simulink model "esercizio2sim_controllore_ricostruttore"  (R2018a)
settings: Solver=VariableStepAuto  StartTime=0.0  StopTime=25  RelTol=1e-7
values from neighbouring files (symbols this model uses):
  A = [2 1 -1; -3 -2 -1; -1 1 -4]    [esercizio1mat.m]    (also in esercizio2mat.m = [0 1 0 0; esercizio3mat.m = [1 1 0; -5 -3 0; 2 3 -1])
  B = B(:, 1)    [esercizio2mat.m]
  C = C(1, :)    [esercizio2mat.m]
  D = D(1, 1)    [esercizio2mat.m]
  g = 9.81    [esercizio2mat.m]
  k = acker(A, -b, autovalori); disp(k)    [esercizio1mat.m]    (also in esercizio2mat.m = acker(A, -B, autov_controllore); disp(k))
  L = 1    [esercizio2mat.m]
  l = lT'; disp(l)    [esercizio1mat.m]    (also in esercizio2mat.m)
  m = 1    [esercizio2mat.m]
  M = 10    [esercizio2mat.m]
  x0 = [0 0 pi/3 .0]'    [esercizio2mat.m]
  xhat0 = x0 + [0.01 -0.02 -0.01 0.02]'    [esercizio2mat.m]
settings Model: Creator=Matteo  LastModifiedBy=Matteo

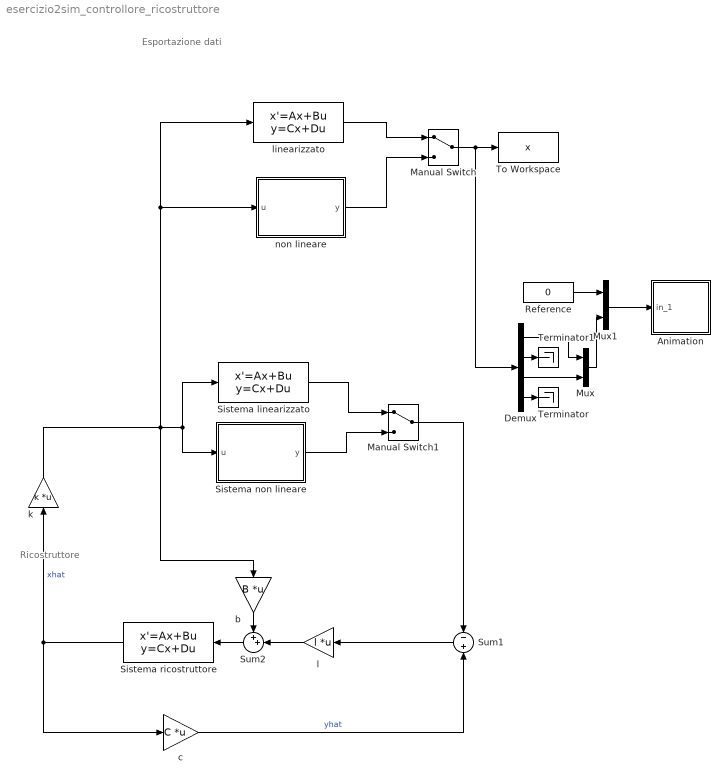
== system esercizio2sim_controllore_ricostruttore ==
  note: Esportazione dati
  note: Ricostruttore
  Animation : Subsystem  mask(Pendulum plot){RefBlock=Reference}
      mask prompts: RefBlock "DC reference signal block name:"
      mask help: Pendulum plot
      mask Help: Pendulum animation function using Handle graphics.
      mask Display: plot([-10 10],[0 0],[-2 -2 2 2],[0 1 1 0],[0 3],[1 5])
  Demux : Demux
  Manual Switch : ManualSwitch
  Manual Switch1 : ManualSwitch
  Mux : Mux  Inputs=2
  Mux1 : Mux  Inputs=2
  Reference : Constant  Value=0
  Sistema linearizzato : StateSpace  A=A  B=B  C=C  D=D  InitialCondition=x0
  Sistema non lineare : Subsystem
  Sistema ricostruttore : StateSpace  A=A  B=eye(4)  C=eye(4)  D=zeros(4)  InitialCondition=xhat0
  Sum1 : Sum  Inputs=-|+
  Sum2 : Sum  Inputs=++|
  Terminator : Terminator
  Terminator1 : Terminator
  To Workspace : ToWorkspace  VariableName=x  SaveFormat=Timeseries  SampleTime=0.05
  b : Gain  Gain=B  Multiplication=Matrix(K*u)
  c : Gain  Gain=C  Multiplication=Matrix(K*u)
  k : Gain  Gain=k  Multiplication=Matrix(K*u)
  l : Gain  Gain=l  Multiplication=Matrix(K*u)
  linearizzato : StateSpace  A=A  B=B  C=eye(4)  D=zeros(4,1)  InitialCondition=x0
  non lineare : Subsystem
  wires:
  Sistema ricostruttore/1 -> c/1, k/1  "xhat"
  Sum1/1 -> l/1
  c/1 -> Sum1/2  "yhat"
  b/1 -> Sum2/1
  l/1 -> Sum2/2
  Sum2/1 -> Sistema ricostruttore/1
  Manual Switch/1 -> Demux/1, To Workspace/1
  linearizzato/1 -> Manual Switch/1
  non lineare/1(y) -> Manual Switch/2
  k/1 -> Sistema non lineare/1(u), Sistema linearizzato/1, b/1, non lineare/1(u), linearizzato/1
  Sistema linearizzato/1 -> Manual Switch1/1
  Manual Switch1/1 -> Sum1/1
  Mux1/1 -> Animation/1(in_1)
  Reference/1 -> Mux1/1
  Demux/2 -> Terminator1/1
  Demux/4 -> Terminator/1
  Demux/1 -> Mux/1
  Demux/3 -> Mux/2
  Mux/1 -> Mux1/2
  Sistema non lineare/1(y) -> Manual Switch1/2

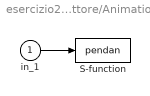
== system esercizio2sim_controllore_ricostruttore/Animation ==
  in_1 : Inport
  S-function : S-Function  FunctionName=pendan  Parameters=RefBlock  SFunctionDeploymentMode=off  EnableBusSupport=off
      settings: DeleteFcn=pendan([],[],[],'DeleteBlock');
  wires:
  in_1/1 -> S-function/1

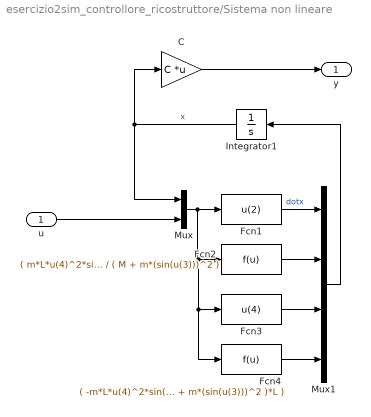
== system esercizio2sim_controllore_ricostruttore/Sistema non lineare ==
  u : Inport
  C : Gain  Gain=C  Multiplication=Matrix(K*u)
  Fcn1 : Fcn  Expr=u(2)
  Fcn2 : Fcn  Expr=( m*L*u(4)^2*sin(u(3)) - m*g*sin(u(3))*cos(u(3)) + u(5) ) / ( M + m*(sin(u(3)))^2 )
  Fcn3 : Fcn  Expr=u(4)
  Fcn4 : Fcn  Expr="( -m*L*u(4)^2*sin(u(3))*cos(u(3)) + (M+m)*g*sin(u(3)) - u(5)*cos(u(3))  ) / ( ( M + m*(sin(u(3)))^2 )*L )"
  Integrator1 : Integrator  InitialCondition=x0
  Mux : Mux  Inputs=2
  Mux1 : Mux
  y : Outport
  wires:
  Fcn2/1 -> Mux1/2
  Fcn1/1 -> Mux1/1  "dotx"
  Fcn3/1 -> Mux1/3
  Fcn4/1 -> Mux1/4
  Mux/1 -> Fcn4/1, Fcn3/1, Fcn2/1, Fcn1/1
  Mux1/1 -> Integrator1/1
  C/1 -> y/1
  Integrator1/1 -> C/1, Mux/1  "x"
  u/1 -> Mux/2

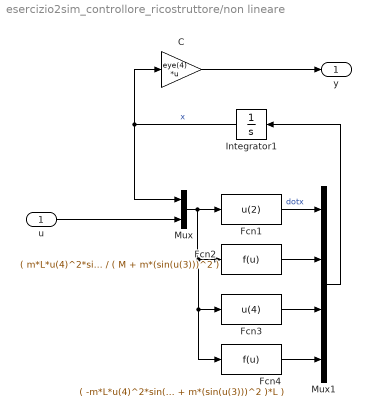
== system esercizio2sim_controllore_ricostruttore/non lineare ==
  u : Inport
  C : Gain  Gain=eye(4)  Multiplication=Matrix(K*u)
  Fcn1 : Fcn  Expr=u(2)
  Fcn2 : Fcn  Expr=( m*L*u(4)^2*sin(u(3)) - m*g*sin(u(3))*cos(u(3)) + u(5) ) / ( M + m*(sin(u(3)))^2 )
  Fcn3 : Fcn  Expr=u(4)
  Fcn4 : Fcn  Expr="( -m*L*u(4)^2*sin(u(3))*cos(u(3)) + (M+m)*g*sin(u(3)) - u(5)*cos(u(3))  ) / ( ( M + m*(sin(u(3)))^2 )*L )"
  Integrator1 : Integrator  InitialCondition=x0
  Mux : Mux  Inputs=2
  Mux1 : Mux
  y : Outport
  wires:
  Integrator1/1 -> C/1, Mux/1  "x"
  Mux/1 -> Fcn4/1, Fcn3/1, Fcn2/1, Fcn1/1
  C/1 -> y/1
  Fcn1/1 -> Mux1/1  "dotx"
  Fcn2/1 -> Mux1/2
  Fcn3/1 -> Mux1/3
  Fcn4/1 -> Mux1/4
  Mux1/1 -> Integrator1/1
  u/1 -> Mux/2
